simulink model "ControleEE"  (R2022b)
settings: Solver=ode45  StartTime=0.0  StopTime=40  RelTol=1e-6  EnableMultiTasking=on
values from neighbouring files (symbols this model uses):
  K = acker(A,B,p)    [PrObsPertContinuoRed.m]    (also in PrPara2nl_PI.m = acker(Aa,Ba,[p,p,p]); TestesEE.m = acker(A,B,[p,p,p]); TestesEEcanalI.m = acker(A,B,[p,-.6-1.0198i,-.6+1.0198i]); TestesEEobsPert.m = acker(A,B,[p,-.6-1.0198i,-.6+1.0198i]))
  L = L'    [PrObsPertContinuoRed.m]    (also in PrPara2nl_PI.m; TestesEE.m; TestesEEcanalI.m; TestesEEobsPert.m)
  Nb = gf.den{1}(1,2)/gf.num{1}(1,2)    [PrObsPertContinuoRed.m]    (also in PrPara2nl_PI.m = gf.den{1}(1,3)/gf.num{1}(1,3); TestesEE.m = gf.den{1}(1,4)/gf.num{1}(1,4); TestesEEcanalI.m = gf.den{1}(1,4)/gf.num{1}(1,4); TestesEEobsPert.m = gf.den{1}(1,4)/gf.num{1}(1,4))
settings Model: Creator=Adolfo  LastModifiedBy=adolfo
settings SolverCC: AlgebraicLoopSolver=TrustRegion
settings DataIOCC: LimitDataPoints=on  SaveFormat=Array  SignalLoggingSaveFormat=ModelDataLogs  ReturnWorkspaceOutputs=off
settings OptimizationCC: ExpressionDepthLimit=2147483647  InitFltsAndDblsToZero=on  LifeSpan=inf
settings DebuggingCC: SaveWithParameterizedLinksMsg=none  UnderspecifiedInitializationDetection=Classic  MergeDetectMultiDrivingBlocksExec=none  SignalResolutionControl=TryResolveAllWithWarning  SolverPrmCheckMsg=warning  MultiTaskDSMMsg=warning  MultiTaskCondExecSysMsg=none  FcnCallInpInsideContextMsg=warning  UnconnectedInputMsg=warning  UnconnectedOutputMsg=warning  UnconnectedLineMsg=warning  StateNameClashWarn=warning  SFUnexpectedBacktrackingDiag=warning  SFNoUnconditionalDefaultTransitionDiag=warning  SFExecutionAtInitializationDiag=none  SFMachineParentedDataDiag=warning  ArithmeticOperatorsInVariantConditions=warning
settings HardwareCC: ProdBitPerPointer=32  ProdBitPerSizeT=32  ProdBitPerPtrDiffT=32  ProdLargestAtomicFloat=None  ProdIntDivRoundTo=Undefined  ProdEndianess=Unspecified  ProdWordSize=32  ProdHWDeviceType=32-bit Generic
settings ModelReferenceCC: EnableRefExpFcnMdlSchedulingChecks=on  PropagateSignalLabelsOutOfModel=off
settings SFSimCC: SimUseLocalCustomCode=off  CustomCodeUndefinedFunction=UseInterfaceOnly
settings RTWCC: RTWUseLocalCustomCode=off
settings CodeAppCC: StateflowObjectComments=on
settings GRTTargetCC: TargetFcnLib=ansi_tfl_tmw.mat  TargetLangStandard=C89/C90 (ANSI)  CombineOutputUpdateFcns=off  GRTInterface=on
settings ConfigComp: CovMetricSettings=dw  CovSaveCumulativeToWorkspaceVar=on  CovSaveSingleToWorkspaceVar=on  CovExternalEMLEnable=off

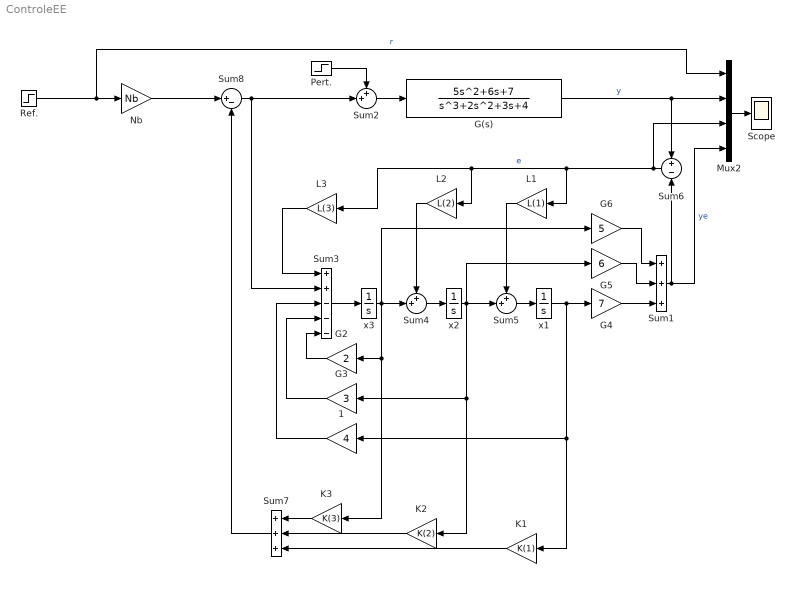
== system ControleEE ==
  1 : Gain  Gain=4
  G(s) : TransferFcn  Numerator=[5 6 7]  Denominator=[1 2 3 4]
  G2 : Gain  Gain=2
  G3 : Gain  Gain=3
  G4 : Gain  Gain=7
  G5 : Gain  Gain=6
  G6 : Gain  Gain=5
  K1 : Gain  Gain=K(1)
  K2 : Gain  Gain=K(2)
  K3 : Gain  Gain=K(3)
  L1 : Gain  Gain=L(1)
  L2 : Gain  Gain=L(2)
  L3 : Gain  Gain=L(3)
  Mux2 : Mux
  Nb : Gain  Gain=Nb
  Pert. : Step  Time=10  SampleTime=0
  Ref. : Step  Time=5  SampleTime=0
  Scope : Scope
  Sum1 : Sum  Inputs=+++
  Sum2 : Sum  Inputs=++|
  Sum3 : Sum  Inputs=++---
  Sum4 : Sum  Inputs=++|
  Sum5 : Sum  Inputs=++|
  Sum6 : Sum  Inputs=+-
  Sum7 : Sum  Inputs=+++
  Sum8 : Sum  Inputs=|+-
  x1 : Integrator
  x2 : Integrator
  x3 : Integrator
  wires:
  Ref./1 -> Mux2/1, Nb/1  "r"
  Mux2/1 -> Scope/1
  x3/1 -> G6/1, Sum4/2, G2/1, K3/1
  x2/1 -> G5/1, Sum5/2, G3/1, K2/1
  Sum3/1 -> x3/1
  G2/1 -> Sum3/5
  G3/1 -> Sum3/4
  x1/1 -> G4/1, 1/1, K1/1
  1/1 -> Sum3/3
  G4/1 -> Sum1/3
  G5/1 -> Sum1/2
  G6/1 -> Sum1/1
  G(s)/1 -> Mux2/2, Sum6/1  "y"
  Sum1/1 -> Sum6/2, Mux2/4  "ye"
  Sum2/1 -> G(s)/1
  Sum4/1 -> x2/1
  Sum5/1 -> x1/1
  L3/1 -> Sum3/1
  L2/1 -> Sum4/1
  L1/1 -> Sum5/1
  K3/1 -> Sum7/1
  K2/1 -> Sum7/2
  K1/1 -> Sum7/3
  Sum8/1 -> Sum3/2, Sum2/2
  Nb/1 -> Sum8/1
  Sum6/1 -> Mux2/3, L3/1, L2/1, L1/1  "e"
  Sum7/1 -> Sum8/2
  Pert./1 -> Sum2/1
